simulink model "test1"  (R2015a)
settings: Solver=ode3  StartTime=0.0  StopTime=10.0  RelTol=1e-3
libraries: PoliArd x6
settings Model: ExtModeTrigDuration=2  Creator=User  LastModifiedBy=dell
settings OptimizationCC: OptimizeModelRefInitCode=on  LifeSpan=1
settings DebuggingCC: UnderspecifiedInitializationDetection=Classic  MergeDetectMultiDrivingBlocksExec=none
settings HardwareCC: ProdLargestAtomicInteger=Long  ProdLargestAtomicFloat=Double  ProdEndianess=LittleEndian  ProdHWDeviceType=ARM Compatible->ARM Cortex
settings RTWCC: SystemTargetFile=realtime.tlc  GenerateMakefile=off  TemplateMakefile=realtime.tmf  Description=Run on Target Hardware  RTWVerbose=off
settings ERTTargetCC: CombineOutputUpdateFcns=off  ExtModeTransport=3  ExtModeMexFile=ext_serial_win32_comm_rtt  ExtModeMexArgs=0 1 9600  ERTSrcFileBannerTemplate=realtime_code_template.cgt  ERTHdrFileBannerTemplate=realtime_code_template.cgt  ERTDataSrcFileTemplate=realtime_code_template.cgt  ERTDataHdrFileTemplate=realtime_code_template.cgt  ERTCustomFileTemplate=realtime_file_process.tlc

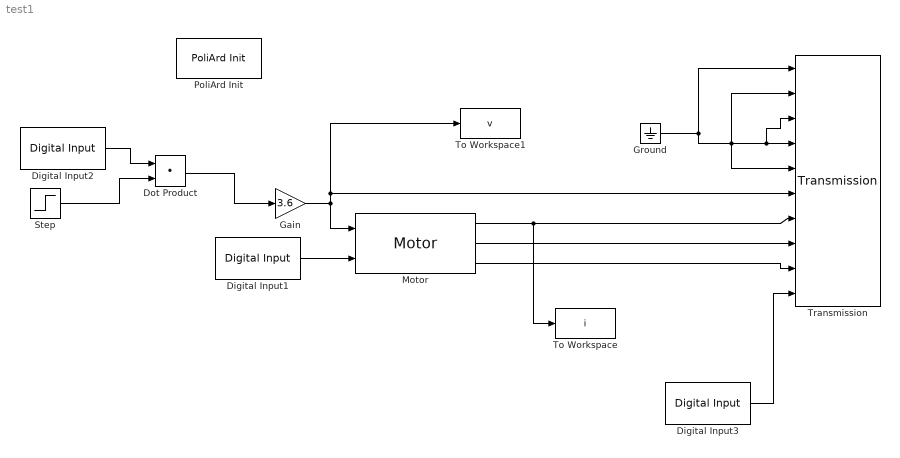
== system test1 ==
  Digital Input1 : PoliArd/Digital Input  DI_pin=3  DIsample=-1
  Digital Input2 : PoliArd/Digital Input  DI_pin=2  DIsample=-1
  Digital Input3 : PoliArd/Digital Input  DI_pin=3  DIsample=-1
  Dot Product : DotProduct  InputSameDT=on  OutDataTypeStr=Inherit: Inherit via internal rule
  Gain : Gain  Gain=3.6
  Ground : Ground
  Motor : PoliArd/Motor  MotorID=1  DC_bus_mask=12  dt_mot=-1
  PoliArd Init : PoliArd/PoliArd Init
  Step : Step  Time=0  SampleTime=0
  To Workspace : ToWorkspace  VariableName=i  SaveFormat=Timeseries  SampleTime=0.0001
  To Workspace1 : ToWorkspace  VariableName=v  SaveFormat=Timeseries  SampleTime=0.0001
  Transmission : PoliArd/Transmission  sample_freq=100  sig_to_send=6
  wires:
  Digital Input1/1 -> Motor/2
  Ground/1 -> Transmission/2, Transmission/5, Transmission/3, Transmission/4, Transmission/1
  Motor/1 -> To Workspace/1, Transmission/7
  Gain/1 -> To Workspace1/1, Transmission/6, Motor/1
  Motor/3 -> Transmission/9
  Motor/2 -> Transmission/8
  Digital Input2/1 -> Dot Product/1
  Step/1 -> Dot Product/2
  Dot Product/1 -> Gain/1
  Digital Input3/1 -> Transmission/10
